simulink model "Channelizer_demo_panel"  (R2023b)
settings: Solver=VariableStepAuto  StartTime=0.0  StopTime=inf  RelTol=1e-3
PostLoadFcn:
  | TT = numerictype(1,16,15);
  | FF = fimath('RoundingMethod','Nearest','OverflowAction','Saturate');
  | mdl = channelizer_init(TT, FF);
  | channelizer = channelizer_model(mdl, TT, FF );
  | Ts = 16*(7/4)/8.75e9;
  | ch_filt_coef = rcosdesign(0.22,4,28,'normal');
  | ch_filt_coef = 28 * ch_filt_coef / sum(ch_filt_coef(:));
  | channelizer_demo_init;
values from neighbouring files (symbols this model uses):
  ch0_en = 0    [channelizer_demo_init.m]    (also in init.m)
  ch0_qam = 0    [channelizer_demo_init.m]    (also in init.m)
  ch0_swp = 0    [channelizer_demo_init.m]    (also in init.m)
  ch10_en = 0    [channelizer_demo_init.m]    (also in init.m)
  ch10_qam = 0    [channelizer_demo_init.m]    (also in init.m)
  ch10_swp = 0    [channelizer_demo_init.m]    (also in init.m)
  ch11_en = 0    [channelizer_demo_init.m]    (also in init.m)
  ch11_qam = 0    [channelizer_demo_init.m]    (also in init.m)
  ch11_swp = 0    [channelizer_demo_init.m]    (also in init.m)
  ch12_en = 0    [channelizer_demo_init.m]    (also in init.m)
  ch12_qam = 0    [channelizer_demo_init.m]    (also in init.m)
  ch12_swp = 0    [channelizer_demo_init.m]    (also in init.m)
  ch13_en = 0    [channelizer_demo_init.m]    (also in init.m)
  ch13_qam = 0    [channelizer_demo_init.m]    (also in init.m)
  ch13_swp = 0    [channelizer_demo_init.m]    (also in init.m)
  ch14_en = 0    [channelizer_demo_init.m]    (also in init.m)
  ch14_qam = 0    [channelizer_demo_init.m]    (also in init.m)
  ch14_swp = 0    [channelizer_demo_init.m]    (also in init.m)
  ch15_en = 0    [channelizer_demo_init.m]    (also in init.m)
  ch15_qam = 0    [channelizer_demo_init.m]    (also in init.m)
  ch15_swp = 0    [channelizer_demo_init.m]    (also in init.m)
  ch1_en = 1    [channelizer_demo_init.m]    (also in init.m)
  ch1_qam = 0    [channelizer_demo_init.m]    (also in init.m)
  ch1_swp = 0    [channelizer_demo_init.m]    (also in init.m)
  ch2_en = 1    [channelizer_demo_init.m]    (also in init.m)
  ch2_qam = 0    [channelizer_demo_init.m]    (also in init.m)
  ch2_swp = 0    [channelizer_demo_init.m]    (also in init.m)
  ch3_en = 0    [channelizer_demo_init.m]    (also in init.m)
  ch3_qam = 0    [channelizer_demo_init.m]    (also in init.m)
  ch3_swp = 0    [channelizer_demo_init.m]    (also in init.m)
  ch4_en = 0    [channelizer_demo_init.m]    (also in init.m)
  ch4_qam = 0    [channelizer_demo_init.m]    (also in init.m)
  ch4_swp = 0    [channelizer_demo_init.m]    (also in init.m)
  ch5_en = 1    [channelizer_demo_init.m]    (also in init.m)
  ch5_qam = 1    [channelizer_demo_init.m]    (also in init.m)
  ch5_swp = 0    [channelizer_demo_init.m]    (also in init.m)
  ch6_en = 1    [channelizer_demo_init.m]    (also in init.m)
  ch6_qam = 1    [channelizer_demo_init.m]    (also in init.m)
  ch6_swp = 0    [channelizer_demo_init.m]    (also in init.m)
  ch7_en = 0    [channelizer_demo_init.m]    (also in init.m)
  ch7_qam = 0    [channelizer_demo_init.m]    (also in init.m)
  ch7_swp = 0    [channelizer_demo_init.m]    (also in init.m)
  ch8_en = 0    [channelizer_demo_init.m]    (also in init.m)
  ch8_qam = 0    [channelizer_demo_init.m]    (also in init.m)
  ch8_swp = 0    [channelizer_demo_init.m]    (also in init.m)
  ch9_en = 0    [channelizer_demo_init.m]    (also in init.m)
  ch9_qam = 0    [channelizer_demo_init.m]    (also in init.m)
  ch9_swp = 0    [channelizer_demo_init.m]    (also in init.m)
  spec1_ch = 1    [channelizer_demo_init.m]    (also in init.m)
  spec2_ch = 2    [channelizer_demo_init.m]    (also in init.m)
  spec3_ch = 5    [channelizer_demo_init.m]    (also in init.m)
  spec4_ch = 6    [channelizer_demo_init.m]    (also in init.m)
  swp_rate0 = 0    [channelizer_demo_init.m]    (also in init.m)
  swp_rate1 = 0    [channelizer_demo_init.m]    (also in init.m)
  swp_rate10 = 0    [channelizer_demo_init.m]    (also in init.m)
  swp_rate11 = 0    [channelizer_demo_init.m]    (also in init.m)
  swp_rate12 = 0    [channelizer_demo_init.m]    (also in init.m)
  swp_rate13 = 0    [channelizer_demo_init.m]    (also in init.m)
  swp_rate14 = 0    [channelizer_demo_init.m]    (also in init.m)
  swp_rate15 = 0    [channelizer_demo_init.m]    (also in init.m)
  swp_rate2 = 0    [channelizer_demo_init.m]    (also in init.m)
  swp_rate3 = 0    [channelizer_demo_init.m]    (also in init.m)
  swp_rate4 = 0    [channelizer_demo_init.m]    (also in init.m)
  swp_rate5 = 0    [channelizer_demo_init.m]    (also in init.m)
  swp_rate6 = 0    [channelizer_demo_init.m]    (also in init.m)
  swp_rate7 = 0    [channelizer_demo_init.m]    (also in init.m)
  swp_rate8 = 0    [channelizer_demo_init.m]    (also in init.m)
  swp_rate9 = 0    [channelizer_demo_init.m]    (also in init.m)
undefined symbols (not defined in the file or in its folder): S, vsva2197, xcvc1902
libraries: aieUtilities x39, aieBasic x34, dspswit3 x16, dspsigops x16, hlsBasic x3, vmcUtilities x1, commchan3 x1
(part 3 of 5)

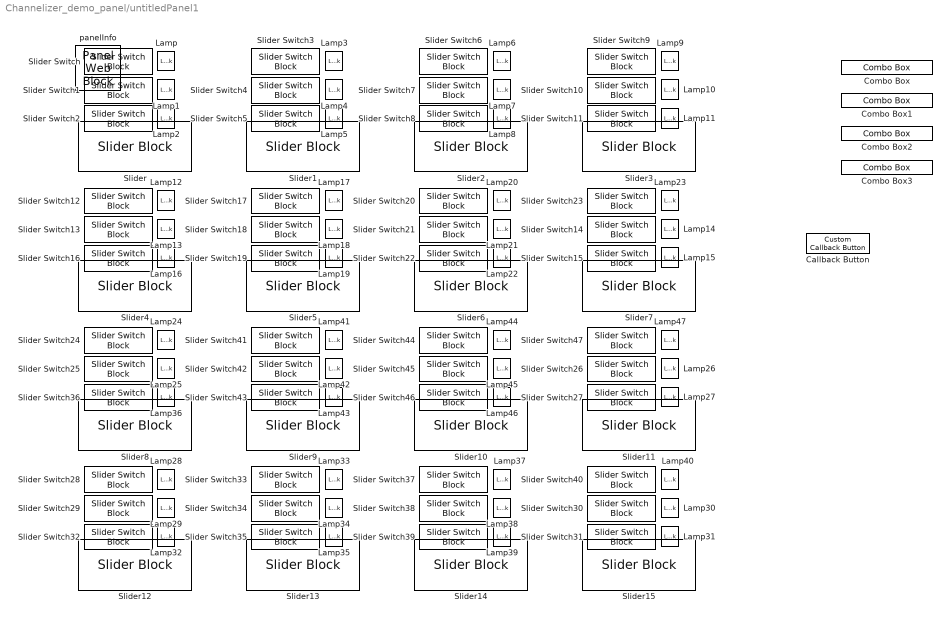
== system Channelizer_demo_panel/untitledPanel1 ==
  Callback Button : CustomCallbackButton  Tag=HiddenForWebPanel  PanelInfo="{\"addnFilesFolder\":\"\",\"height\":22,\"includeDebugPackages\":false,\"left\":833,\"outputFolder\":\"\",\"panelId\":\"panelId-6526f2f6-f2b9-454a-b79d-ddfd0d3181f7\",\"popoutMode\":\"\",\"standaloneTitle\":\"\",\"top\":225,\"type\":\"panelChild\",\"version\":\"2019b\",\"width\":70,\"zIndex\":1500128}"  Configuration="{\"components\":[{\"name\":\"BackgroundImageComponent\",\"settings\":{\"image\":{\"size\":[0,0],\"src\":\"default\",\"srcOrientation\":\"Right\"},\"position\":[0,0,1,1]}},{\"name\":\"ButtonStateComponent\",\"settings\":{\"buttonType\":\"momentary\",\"clickFcn\":\"channelizer_demo_init;\",\"onValue\":1,\"position\":[0,0,1,1],\"pressDelay\":\"500\",\"pressFcn\":\"\",\"repeatInterval\":\"0\",\"states\":[{\"horizontalAlignment\":\"center\",\"image\":{\"position\":[0,0,1,1],\"size\":[1,1],\"src\":\"default\",\"srcOrientation\":\"Right\"},\"label\":{\"color\":[1,1,1],\"icon\":{\"size\":[0,0],\"src\":\"default\",\"srcOrientation\":\"Right\"},\"iconPlacement\":\"left\",\"opacity\":1,\"show\":true,\"text\":{\"content\":\"RESET\",\"font\":\"Helvetica\",\"fontSize\":12}},\"labelOffset\":[0,0],\"verticalAlignment\":\"middle\"},{\"horizontalAlignment\":\"center\",\"image\":{\"position\":[0,0,1,1],\"size\":[1,1],\"src\":\"default\",\"srcOrientation\":\"Right\"},\"label\":{\"color\":[1,1,1],\"icon\":{\"size\":[0,0],\"src\":\"default\",\"srcOrientation\":\"Right\"},\"iconPlacement\":\"left\",\"opacity\":1,\"show\":true,\"text\":{\"content\":\"RESET\",\"font\":\"Helvetica\",\"fontSize\":12}},\"labelOffset\":[0,0],\"verticalAlignment\":\"middle\"},{\"horizontalAlignment\":\"center\",\"image\":{\"position\":[0,0,1,1],\"size\":[1,1],\"src\":\"default\",\"srcOrientation\":\"Right\"},\"label\":{\"color\":[1,1,1],\"icon\":{\"size\":[0,0],\"src\":\"default\",\"srcOrientation\":\"Right\"},\"iconPlacement\":\"left\",\"opacity\":1,\"show\":true,\"text\":{\"content\":\"RESET\",\"font\":\"Helvetica\",\"fontSize\":12}},\"labelOffset\":[0,0],\"verticalAlignment\":\"middle\"},{\"horizontalAlignment\":\"center\",\"image\":{\"position\":[0,0,1,1],\"size\":[1,1],\"src\":\"default\",\"srcOrientation\":\"Right\"},\"label\":{\"color\":[1,1,1],\"icon\":{\"size\":[0,0],\"src\":\"default\",\"srcOrientation\":\"Right\"},\"iconPlacement\":\"left\",\"opacity\":1,\"show\":true,\"text\":{\"content\":\"RESET\",\"font\":\"Helvetica\",\"fontSize\":12}},\"labelOffset\":[0,0],\"verticalAlignment\":\"middle\"}]}},{\"name\":\"ForegroundImageComponent\",\"settings\":{\"image\":{\"size\":[0,0],\"src\":\"default\",\"srcOrientation\":\"Right\"},\"isForeground\":1,\"position\":[0,0,1,1]}}],\"settings\":{\"BindingType\":\"standalone\",\"backgroundColor\":[244,244,244,1],\"backgroundOffset\":0.2,\"backgroundOpacity\":1,\"fixedAspectRatio\":\"on\",\"foregroundColor\":[0.01176470588,0.01176470588,0.01176470588,1],\"migratedFromLegacy\":true,\"useBackgroundColor\":true,\"variant\":\"callback\",\"version\":\"R2023a\"},\"type\":\"Button\"}"  CustomBackgroundColor="{\"color\":[0,0.447059,0.741176],\"show\":true}"
  Combo Box : ComboBox  Tag=HiddenForWebPanel  PanelInfo="{\"addnFilesFolder\":\"\",\"height\":16,\"includeDebugPackages\":false,\"left\":872,\"outputFolder\":\"\",\"panelId\":\"panelId-6526f2f6-f2b9-454a-b79d-ddfd0d3181f7\",\"popoutMode\":\"\",\"standaloneTitle\":\"\",\"top\":31,\"type\":\"panelChild\",\"version\":\"2019b\",\"width\":102,\"zIndex\":1500228}"  LabelPosition=Hide  SelectedLabel=Channel 1
      settings: Values={{'Channel 0', 'Channel 1', 'Channel 2', 'Channel 3', 'Channel 4', 'Channel 5', 'Channel 6', 'Channel 7', 'Channel 8', 'Channel 9', 'Channel 10', 'Channel 11', 'Channel 12', 'Channel 13', 'Channel 14', 'Channel 15'}, [0 1 2 3 4 5 6 7 8 9 10 11 12 13 14 15]}
  Combo Box1 : ComboBox  Tag=HiddenForWebPanel  PanelInfo="{\"addnFilesFolder\":\"\",\"height\":16,\"includeDebugPackages\":false,\"left\":872,\"outputFolder\":\"\",\"panelId\":\"panelId-6526f2f6-f2b9-454a-b79d-ddfd0d3181f7\",\"popoutMode\":\"\",\"standaloneTitle\":\"\",\"top\":68,\"type\":\"panelChild\",\"version\":\"2019b\",\"width\":102,\"zIndex\":1500208}"  LabelPosition=Hide  SelectedLabel=Channel 2
      settings: Values={{'Channel 0', 'Channel 1', 'Channel 2', 'Channel 3', 'Channel 4', 'Channel 5', 'Channel 6', 'Channel 7', 'Channel 8', 'Channel 9', 'Channel 10', 'Channel 11', 'Channel 12', 'Channel 13', 'Channel 14', 'Channel 15'}, [0 1 2 3 4 5 6 7 8 9 10 11 12 13 14 15]}
  Combo Box2 : ComboBox  Tag=HiddenForWebPanel  PanelInfo="{\"addnFilesFolder\":\"\",\"height\":16,\"includeDebugPackages\":false,\"left\":872,\"outputFolder\":\"\",\"panelId\":\"panelId-6526f2f6-f2b9-454a-b79d-ddfd0d3181f7\",\"popoutMode\":\"\",\"standaloneTitle\":\"\",\"top\":105,\"type\":\"panelChild\",\"version\":\"2019b\",\"width\":102,\"zIndex\":1500198}"  LabelPosition=Hide  SelectedLabel=Channel 5
      settings: Values={{'Channel 0', 'Channel 1', 'Channel 2', 'Channel 3', 'Channel 4', 'Channel 5', 'Channel 6', 'Channel 7', 'Channel 8', 'Channel 9', 'Channel 10', 'Channel 11', 'Channel 12', 'Channel 13', 'Channel 14', 'Channel 15'}, [0 1 2 3 4 5 6 7 8 9 10 11 12 13 14 15]}
  Combo Box3 : ComboBox  Tag=HiddenForWebPanel  PanelInfo="{\"addnFilesFolder\":\"\",\"height\":16,\"includeDebugPackages\":false,\"left\":872,\"outputFolder\":\"\",\"panelId\":\"panelId-6526f2f6-f2b9-454a-b79d-ddfd0d3181f7\",\"popoutMode\":\"\",\"standaloneTitle\":\"\",\"top\":143,\"type\":\"panelChild\",\"version\":\"2019b\",\"width\":102,\"zIndex\":1500096}"  LabelPosition=Hide  SelectedLabel=Channel 6
      settings: Values={{'Channel 0', 'Channel 1', 'Channel 2', 'Channel 3', 'Channel 4', 'Channel 5', 'Channel 6', 'Channel 7', 'Channel 8', 'Channel 9', 'Channel 10', 'Channel 11', 'Channel 12', 'Channel 13', 'Channel 14', 'Channel 15'}, [0 1 2 3 4 5 6 7 8 9 10 11 12 13 14 15]}
  Lamp : LampBlock  Tag=HiddenForWebPanel  PanelInfo="{\"addnFilesFolder\":\"\",\"height\":22,\"includeDebugPackages\":false,\"left\":107,\"outputFolder\":\"\",\"panelId\":\"panelId-6526f2f6-f2b9-454a-b79d-ddfd0d3181f7\",\"popoutMode\":\"\",\"standaloneTitle\":\"\",\"top\":21,\"type\":\"panelChild\",\"version\":\"2019b\",\"width\":19,\"zIndex\":1500094}"  LabelPosition=Hide
  Lamp1 : LampBlock  Tag=HiddenForWebPanel  PanelInfo="{\"addnFilesFolder\":\"\",\"height\":22,\"includeDebugPackages\":false,\"left\":107,\"outputFolder\":\"\",\"panelId\":\"panelId-6526f2f6-f2b9-454a-b79d-ddfd0d3181f7\",\"popoutMode\":\"\",\"standaloneTitle\":\"\",\"top\":53,\"type\":\"panelChild\",\"version\":\"2019b\",\"width\":19,\"zIndex\":1500030}"  LabelPosition=Hide
  Lamp10 : LampBlock  Tag=HiddenForWebPanel  PanelInfo="{\"addnFilesFolder\":\"\",\"height\":22,\"includeDebugPackages\":false,\"left\":671,\"outputFolder\":\"\",\"panelId\":\"panelId-6526f2f6-f2b9-454a-b79d-ddfd0d3181f7\",\"popoutMode\":\"\",\"standaloneTitle\":\"\",\"top\":53,\"type\":\"panelChild\",\"version\":\"2019b\",\"width\":19,\"zIndex\":1500212}"  LabelPosition=Hide
  Lamp11 : LampBlock  Tag=HiddenForWebPanel  PanelInfo="{\"addnFilesFolder\":\"\",\"height\":22,\"includeDebugPackages\":false,\"left\":671,\"outputFolder\":\"\",\"panelId\":\"panelId-6526f2f6-f2b9-454a-b79d-ddfd0d3181f7\",\"popoutMode\":\"\",\"standaloneTitle\":\"\",\"top\":85,\"type\":\"panelChild\",\"version\":\"2019b\",\"width\":19,\"zIndex\":1500102}"  LabelPosition=Hide
  Lamp12 : LampBlock  Tag=HiddenForWebPanel  PanelInfo="{\"addnFilesFolder\":\"\",\"height\":22,\"includeDebugPackages\":false,\"left\":107,\"outputFolder\":\"\",\"panelId\":\"panelId-6526f2f6-f2b9-454a-b79d-ddfd0d3181f7\",\"popoutMode\":\"\",\"standaloneTitle\":\"\",\"top\":177,\"type\":\"panelChild\",\"version\":\"2019b\",\"width\":19,\"zIndex\":1500110}"  LabelPosition=Hide
  Lamp13 : LampBlock  Tag=HiddenForWebPanel  PanelInfo="{\"addnFilesFolder\":\"\",\"height\":22,\"includeDebugPackages\":false,\"left\":107,\"outputFolder\":\"\",\"panelId\":\"panelId-6526f2f6-f2b9-454a-b79d-ddfd0d3181f7\",\"popoutMode\":\"\",\"standaloneTitle\":\"\",\"top\":209,\"type\":\"panelChild\",\"version\":\"2019b\",\"width\":19,\"zIndex\":1500034}"  LabelPosition=Hide
  Lamp14 : LampBlock  Tag=HiddenForWebPanel  PanelInfo="{\"addnFilesFolder\":\"\",\"height\":22,\"includeDebugPackages\":false,\"left\":671,\"outputFolder\":\"\",\"panelId\":\"panelId-6526f2f6-f2b9-454a-b79d-ddfd0d3181f7\",\"popoutMode\":\"\",\"standaloneTitle\":\"\",\"top\":209,\"type\":\"panelChild\",\"version\":\"2019b\",\"width\":19,\"zIndex\":1500166}"  LabelPosition=Hide
  Lamp15 : LampBlock  Tag=HiddenForWebPanel  PanelInfo="{\"addnFilesFolder\":\"\",\"height\":22,\"includeDebugPackages\":false,\"left\":671,\"outputFolder\":\"\",\"panelId\":\"panelId-6526f2f6-f2b9-454a-b79d-ddfd0d3181f7\",\"popoutMode\":\"\",\"standaloneTitle\":\"\",\"top\":241,\"type\":\"panelChild\",\"version\":\"2019b\",\"width\":19,\"zIndex\":1500042}"  LabelPosition=Hide
  Lamp16 : LampBlock  Tag=HiddenForWebPanel  PanelInfo="{\"addnFilesFolder\":\"\",\"height\":22,\"includeDebugPackages\":false,\"left\":107,\"outputFolder\":\"\",\"panelId\":\"panelId-6526f2f6-f2b9-454a-b79d-ddfd0d3181f7\",\"popoutMode\":\"\",\"standaloneTitle\":\"\",\"top\":241,\"type\":\"panelChild\",\"version\":\"2019b\",\"width\":19,\"zIndex\":1500210}"  LabelPosition=Hide
  Lamp17 : LampBlock  Tag=HiddenForWebPanel  PanelInfo="{\"addnFilesFolder\":\"\",\"height\":22,\"includeDebugPackages\":false,\"left\":295,\"outputFolder\":\"\",\"panelId\":\"panelId-6526f2f6-f2b9-454a-b79d-ddfd0d3181f7\",\"popoutMode\":\"\",\"standaloneTitle\":\"\",\"top\":177,\"type\":\"panelChild\",\"version\":\"2019b\",\"width\":19,\"zIndex\":1500108}"  LabelPosition=Hide
  Lamp18 : LampBlock  Tag=HiddenForWebPanel  PanelInfo="{\"addnFilesFolder\":\"\",\"height\":22,\"includeDebugPackages\":false,\"left\":295,\"outputFolder\":\"\",\"panelId\":\"panelId-6526f2f6-f2b9-454a-b79d-ddfd0d3181f7\",\"popoutMode\":\"\",\"standaloneTitle\":\"\",\"top\":209,\"type\":\"panelChild\",\"version\":\"2019b\",\"width\":19,\"zIndex\":1500200}"  LabelPosition=Hide
  Lamp19 : LampBlock  Tag=HiddenForWebPanel  PanelInfo="{\"addnFilesFolder\":\"\",\"height\":22,\"includeDebugPackages\":false,\"left\":295,\"outputFolder\":\"\",\"panelId\":\"panelId-6526f2f6-f2b9-454a-b79d-ddfd0d3181f7\",\"popoutMode\":\"\",\"standaloneTitle\":\"\",\"top\":241,\"type\":\"panelChild\",\"version\":\"2019b\",\"width\":19,\"zIndex\":1500188}"  LabelPosition=Hide
  Lamp2 : LampBlock  Tag=HiddenForWebPanel  PanelInfo="{\"addnFilesFolder\":\"\",\"height\":22,\"includeDebugPackages\":false,\"left\":107,\"outputFolder\":\"\",\"panelId\":\"panelId-6526f2f6-f2b9-454a-b79d-ddfd0d3181f7\",\"popoutMode\":\"\",\"standaloneTitle\":\"\",\"top\":85,\"type\":\"panelChild\",\"version\":\"2019b\",\"width\":19,\"zIndex\":1500028}"  LabelPosition=Hide
  Lamp20 : LampBlock  Tag=HiddenForWebPanel  PanelInfo="{\"addnFilesFolder\":\"\",\"height\":22,\"includeDebugPackages\":false,\"left\":483,\"outputFolder\":\"\",\"panelId\":\"panelId-6526f2f6-f2b9-454a-b79d-ddfd0d3181f7\",\"popoutMode\":\"\",\"standaloneTitle\":\"\",\"top\":177,\"type\":\"panelChild\",\"version\":\"2019b\",\"width\":19,\"zIndex\":1500116}"  LabelPosition=Hide
  Lamp21 : LampBlock  Tag=HiddenForWebPanel  PanelInfo="{\"addnFilesFolder\":\"\",\"height\":22,\"includeDebugPackages\":false,\"left\":483,\"outputFolder\":\"\",\"panelId\":\"panelId-6526f2f6-f2b9-454a-b79d-ddfd0d3181f7\",\"popoutMode\":\"\",\"standaloneTitle\":\"\",\"top\":209,\"type\":\"panelChild\",\"version\":\"2019b\",\"width\":19,\"zIndex\":1500072}"  LabelPosition=Hide
  Lamp22 : LampBlock  Tag=HiddenForWebPanel  PanelInfo="{\"addnFilesFolder\":\"\",\"height\":22,\"includeDebugPackages\":false,\"left\":483,\"outputFolder\":\"\",\"panelId\":\"panelId-6526f2f6-f2b9-454a-b79d-ddfd0d3181f7\",\"popoutMode\":\"\",\"standaloneTitle\":\"\",\"top\":241,\"type\":\"panelChild\",\"version\":\"2019b\",\"width\":19,\"zIndex\":1500046}"  LabelPosition=Hide
  Lamp23 : LampBlock  Tag=HiddenForWebPanel  PanelInfo="{\"addnFilesFolder\":\"\",\"height\":22,\"includeDebugPackages\":false,\"left\":671,\"outputFolder\":\"\",\"panelId\":\"panelId-6526f2f6-f2b9-454a-b79d-ddfd0d3181f7\",\"popoutMode\":\"\",\"standaloneTitle\":\"\",\"top\":177,\"type\":\"panelChild\",\"version\":\"2019b\",\"width\":19,\"zIndex\":1500004}"  LabelPosition=Hide
  Lamp24 : LampBlock  Tag=HiddenForWebPanel  PanelInfo="{\"addnFilesFolder\":\"\",\"height\":22,\"includeDebugPackages\":false,\"left\":107,\"outputFolder\":\"\",\"panelId\":\"panelId-6526f2f6-f2b9-454a-b79d-ddfd0d3181f7\",\"popoutMode\":\"\",\"standaloneTitle\":\"\",\"top\":333,\"type\":\"panelChild\",\"version\":\"2019b\",\"width\":19,\"zIndex\":1500078}"  LabelPosition=Hide
  Lamp25 : LampBlock  Tag=HiddenForWebPanel  PanelInfo="{\"addnFilesFolder\":\"\",\"height\":22,\"includeDebugPackages\":false,\"left\":107,\"outputFolder\":\"\",\"panelId\":\"panelId-6526f2f6-f2b9-454a-b79d-ddfd0d3181f7\",\"popoutMode\":\"\",\"standaloneTitle\":\"\",\"top\":365,\"type\":\"panelChild\",\"version\":\"2019b\",\"width\":19,\"zIndex\":1500038}"  LabelPosition=Hide
  Lamp26 : LampBlock  Tag=HiddenForWebPanel  PanelInfo="{\"addnFilesFolder\":\"\",\"height\":22,\"includeDebugPackages\":false,\"left\":671,\"outputFolder\":\"\",\"panelId\":\"panelId-6526f2f6-f2b9-454a-b79d-ddfd0d3181f7\",\"popoutMode\":\"\",\"standaloneTitle\":\"\",\"top\":365,\"type\":\"panelChild\",\"version\":\"2019b\",\"width\":19,\"zIndex\":1500158}"  LabelPosition=Hide
  Lamp27 : LampBlock  Tag=HiddenForWebPanel  PanelInfo="{\"addnFilesFolder\":\"\",\"height\":22,\"includeDebugPackages\":false,\"left\":671,\"outputFolder\":\"\",\"panelId\":\"panelId-6526f2f6-f2b9-454a-b79d-ddfd0d3181f7\",\"popoutMode\":\"\",\"standaloneTitle\":\"\",\"top\":397,\"type\":\"panelChild\",\"version\":\"2019b\",\"width\":19,\"zIndex\":1500024}"  LabelPosition=Hide
  Lamp28 : LampBlock  Tag=HiddenForWebPanel  PanelInfo="{\"addnFilesFolder\":\"\",\"height\":22,\"includeDebugPackages\":false,\"left\":107,\"outputFolder\":\"\",\"panelId\":\"panelId-6526f2f6-f2b9-454a-b79d-ddfd0d3181f7\",\"popoutMode\":\"\",\"standaloneTitle\":\"\",\"top\":489,\"type\":\"panelChild\",\"version\":\"2019b\",\"width\":19,\"zIndex\":1500134}"  LabelPosition=Hide
  Lamp29 : LampBlock  Tag=HiddenForWebPanel  PanelInfo="{\"addnFilesFolder\":\"\",\"height\":22,\"includeDebugPackages\":false,\"left\":107,\"outputFolder\":\"\",\"panelId\":\"panelId-6526f2f6-f2b9-454a-b79d-ddfd0d3181f7\",\"popoutMode\":\"\",\"standaloneTitle\":\"\",\"top\":521,\"type\":\"panelChild\",\"version\":\"2019b\",\"width\":19,\"zIndex\":1500080}"  LabelPosition=Hide
  Lamp3 : LampBlock  Tag=HiddenForWebPanel  PanelInfo="{\"addnFilesFolder\":\"\",\"height\":22,\"includeDebugPackages\":false,\"left\":295,\"outputFolder\":\"\",\"panelId\":\"panelId-6526f2f6-f2b9-454a-b79d-ddfd0d3181f7\",\"popoutMode\":\"\",\"standaloneTitle\":\"\",\"top\":21,\"type\":\"panelChild\",\"version\":\"2019b\",\"width\":19,\"zIndex\":1500056}"  LabelPosition=Hide
  Lamp30 : LampBlock  Tag=HiddenForWebPanel  PanelInfo="{\"addnFilesFolder\":\"\",\"height\":22,\"includeDebugPackages\":false,\"left\":671,\"outputFolder\":\"\",\"panelId\":\"panelId-6526f2f6-f2b9-454a-b79d-ddfd0d3181f7\",\"popoutMode\":\"\",\"standaloneTitle\":\"\",\"top\":521,\"type\":\"panelChild\",\"version\":\"2019b\",\"width\":19,\"zIndex\":1500186}"  LabelPosition=Hide
  Lamp31 : LampBlock  Tag=HiddenForWebPanel  PanelInfo="{\"addnFilesFolder\":\"\",\"height\":22,\"includeDebugPackages\":false,\"left\":671,\"outputFolder\":\"\",\"panelId\":\"panelId-6526f2f6-f2b9-454a-b79d-ddfd0d3181f7\",\"popoutMode\":\"\",\"standaloneTitle\":\"\",\"top\":553,\"type\":\"panelChild\",\"version\":\"2019b\",\"width\":19,\"zIndex\":1500050}"  LabelPosition=Hide
  Lamp32 : LampBlock  Tag=HiddenForWebPanel  PanelInfo="{\"addnFilesFolder\":\"\",\"height\":22,\"includeDebugPackages\":false,\"left\":107,\"outputFolder\":\"\",\"panelId\":\"panelId-6526f2f6-f2b9-454a-b79d-ddfd0d3181f7\",\"popoutMode\":\"\",\"standaloneTitle\":\"\",\"top\":553,\"type\":\"panelChild\",\"version\":\"2019b\",\"width\":19,\"zIndex\":1500088}"  LabelPosition=Hide
  Lamp33 : LampBlock  Tag=HiddenForWebPanel  PanelInfo="{\"addnFilesFolder\":\"\",\"height\":22,\"includeDebugPackages\":false,\"left\":295,\"outputFolder\":\"\",\"panelId\":\"panelId-6526f2f6-f2b9-454a-b79d-ddfd0d3181f7\",\"popoutMode\":\"\",\"standaloneTitle\":\"\",\"top\":489,\"type\":\"panelChild\",\"version\":\"2019b\",\"width\":19,\"zIndex\":1500086}"  LabelPosition=Hide
  Lamp34 : LampBlock  Tag=HiddenForWebPanel  PanelInfo="{\"addnFilesFolder\":\"\",\"height\":22,\"includeDebugPackages\":false,\"left\":295,\"outputFolder\":\"\",\"panelId\":\"panelId-6526f2f6-f2b9-454a-b79d-ddfd0d3181f7\",\"popoutMode\":\"\",\"standaloneTitle\":\"\",\"top\":521,\"type\":\"panelChild\",\"version\":\"2019b\",\"width\":19,\"zIndex\":1500098}"  LabelPosition=Hide
  Lamp35 : LampBlock  Tag=HiddenForWebPanel  PanelInfo="{\"addnFilesFolder\":\"\",\"height\":22,\"includeDebugPackages\":false,\"left\":295,\"outputFolder\":\"\",\"panelId\":\"panelId-6526f2f6-f2b9-454a-b79d-ddfd0d3181f7\",\"popoutMode\":\"\",\"standaloneTitle\":\"\",\"top\":553,\"type\":\"panelChild\",\"version\":\"2019b\",\"width\":19,\"zIndex\":1500100}"  LabelPosition=Hide
  Lamp36 : LampBlock  Tag=HiddenForWebPanel  PanelInfo="{\"addnFilesFolder\":\"\",\"height\":22,\"includeDebugPackages\":false,\"left\":107,\"outputFolder\":\"\",\"panelId\":\"panelId-6526f2f6-f2b9-454a-b79d-ddfd0d3181f7\",\"popoutMode\":\"\",\"standaloneTitle\":\"\",\"top\":397,\"type\":\"panelChild\",\"version\":\"2019b\",\"width\":19,\"zIndex\":1500140}"  LabelPosition=Hide
  Lamp37 : LampBlock  Tag=HiddenForWebPanel  PanelInfo="{\"addnFilesFolder\":\"\",\"height\":22,\"includeDebugPackages\":false,\"left\":483,\"outputFolder\":\"\",\"panelId\":\"panelId-6526f2f6-f2b9-454a-b79d-ddfd0d3181f7\",\"popoutMode\":\"\",\"standaloneTitle\":\"\",\"top\":489,\"type\":\"panelChild\",\"version\":\"2019b\",\"width\":19,\"zIndex\":1500138}"  LabelPosition=Hide
  Lamp38 : LampBlock  Tag=HiddenForWebPanel  PanelInfo="{\"addnFilesFolder\":\"\",\"height\":22,\"includeDebugPackages\":false,\"left\":483,\"outputFolder\":\"\",\"panelId\":\"panelId-6526f2f6-f2b9-454a-b79d-ddfd0d3181f7\",\"popoutMode\":\"\",\"standaloneTitle\":\"\",\"top\":521,\"type\":\"panelChild\",\"version\":\"2019b\",\"width\":19,\"zIndex\":1500206}"  LabelPosition=Hide
  Lamp39 : LampBlock  Tag=HiddenForWebPanel  PanelInfo="{\"addnFilesFolder\":\"\",\"height\":22,\"includeDebugPackages\":false,\"left\":483,\"outputFolder\":\"\",\"panelId\":\"panelId-6526f2f6-f2b9-454a-b79d-ddfd0d3181f7\",\"popoutMode\":\"\",\"standaloneTitle\":\"\",\"top\":553,\"type\":\"panelChild\",\"version\":\"2019b\",\"width\":19,\"zIndex\":1500130}"  LabelPosition=Hide
  Lamp4 : LampBlock  Tag=HiddenForWebPanel  PanelInfo="{\"addnFilesFolder\":\"\",\"height\":22,\"includeDebugPackages\":false,\"left\":295,\"outputFolder\":\"\",\"panelId\":\"panelId-6526f2f6-f2b9-454a-b79d-ddfd0d3181f7\",\"popoutMode\":\"\",\"standaloneTitle\":\"\",\"top\":53,\"type\":\"panelChild\",\"version\":\"2019b\",\"width\":19,\"zIndex\":1500054}"  LabelPosition=Hide
  Lamp40 : LampBlock  Tag=HiddenForWebPanel  PanelInfo="{\"addnFilesFolder\":\"\",\"height\":22,\"includeDebugPackages\":false,\"left\":671,\"outputFolder\":\"\",\"panelId\":\"panelId-6526f2f6-f2b9-454a-b79d-ddfd0d3181f7\",\"popoutMode\":\"\",\"standaloneTitle\":\"\",\"top\":489,\"type\":\"panelChild\",\"version\":\"2019b\",\"width\":19,\"zIndex\":1500016}"  LabelPosition=Hide
  Lamp41 : LampBlock  Tag=HiddenForWebPanel  PanelInfo="{\"addnFilesFolder\":\"\",\"height\":22,\"includeDebugPackages\":false,\"left\":295,\"outputFolder\":\"\",\"panelId\":\"panelId-6526f2f6-f2b9-454a-b79d-ddfd0d3181f7\",\"popoutMode\":\"\",\"standaloneTitle\":\"\",\"top\":333,\"type\":\"panelChild\",\"version\":\"2019b\",\"width\":19,\"zIndex\":1500068}"  LabelPosition=Hide
  Lamp42 : LampBlock  Tag=HiddenForWebPanel  PanelInfo="{\"addnFilesFolder\":\"\",\"height\":22,\"includeDebugPackages\":false,\"left\":295,\"outputFolder\":\"\",\"panelId\":\"panelId-6526f2f6-f2b9-454a-b79d-ddfd0d3181f7\",\"popoutMode\":\"\",\"standaloneTitle\":\"\",\"top\":365,\"type\":\"panelChild\",\"version\":\"2019b\",\"width\":19,\"zIndex\":1500076}"  LabelPosition=Hide
  Lamp43 : LampBlock  Tag=HiddenForWebPanel  PanelInfo="{\"addnFilesFolder\":\"\",\"height\":22,\"includeDebugPackages\":false,\"left\":295,\"outputFolder\":\"\",\"panelId\":\"panelId-6526f2f6-f2b9-454a-b79d-ddfd0d3181f7\",\"popoutMode\":\"\",\"standaloneTitle\":\"\",\"top\":397,\"type\":\"panelChild\",\"version\":\"2019b\",\"width\":19,\"zIndex\":1500084}"  LabelPosition=Hide
  Lamp44 : LampBlock  Tag=HiddenForWebPanel  PanelInfo="{\"addnFilesFolder\":\"\",\"height\":22,\"includeDebugPackages\":false,\"left\":483,\"outputFolder\":\"\",\"panelId\":\"panelId-6526f2f6-f2b9-454a-b79d-ddfd0d3181f7\",\"popoutMode\":\"\",\"standaloneTitle\":\"\",\"top\":333,\"type\":\"panelChild\",\"version\":\"2019b\",\"width\":19,\"zIndex\":1500124}"  LabelPosition=Hide
  Lamp45 : LampBlock  Tag=HiddenForWebPanel  PanelInfo="{\"addnFilesFolder\":\"\",\"height\":22,\"includeDebugPackages\":false,\"left\":483,\"outputFolder\":\"\",\"panelId\":\"panelId-6526f2f6-f2b9-454a-b79d-ddfd0d3181f7\",\"popoutMode\":\"\",\"standaloneTitle\":\"\",\"top\":365,\"type\":\"panelChild\",\"version\":\"2019b\",\"width\":19,\"zIndex\":1500164}"  LabelPosition=Hide
  Lamp46 : LampBlock  Tag=HiddenForWebPanel  PanelInfo="{\"addnFilesFolder\":\"\",\"height\":22,\"includeDebugPackages\":false,\"left\":483,\"outputFolder\":\"\",\"panelId\":\"panelId-6526f2f6-f2b9-454a-b79d-ddfd0d3181f7\",\"popoutMode\":\"\",\"standaloneTitle\":\"\",\"top\":397,\"type\":\"panelChild\",\"version\":\"2019b\",\"width\":19,\"zIndex\":1500132}"  LabelPosition=Hide
  Lamp47 : LampBlock  Tag=HiddenForWebPanel  PanelInfo="{\"addnFilesFolder\":\"\",\"height\":22,\"includeDebugPackages\":false,\"left\":671,\"outputFolder\":\"\",\"panelId\":\"panelId-6526f2f6-f2b9-454a-b79d-ddfd0d3181f7\",\"popoutMode\":\"\",\"standaloneTitle\":\"\",\"top\":333,\"type\":\"panelChild\",\"version\":\"2019b\",\"width\":19,\"zIndex\":1500126}"  LabelPosition=Hide
  Lamp5 : LampBlock  Tag=HiddenForWebPanel  PanelInfo="{\"addnFilesFolder\":\"\",\"height\":22,\"includeDebugPackages\":false,\"left\":295,\"outputFolder\":\"\",\"panelId\":\"panelId-6526f2f6-f2b9-454a-b79d-ddfd0d3181f7\",\"popoutMode\":\"\",\"standaloneTitle\":\"\",\"top\":85,\"type\":\"panelChild\",\"version\":\"2019b\",\"width\":19,\"zIndex\":1500022}"  LabelPosition=Hide
  Lamp6 : LampBlock  Tag=HiddenForWebPanel  PanelInfo="{\"addnFilesFolder\":\"\",\"height\":22,\"includeDebugPackages\":false,\"left\":483,\"outputFolder\":\"\",\"panelId\":\"panelId-6526f2f6-f2b9-454a-b79d-ddfd0d3181f7\",\"popoutMode\":\"\",\"standaloneTitle\":\"\",\"top\":21,\"type\":\"panelChild\",\"version\":\"2019b\",\"width\":19,\"zIndex\":1500044}"  LabelPosition=Hide
  Lamp7 : LampBlock  Tag=HiddenForWebPanel  PanelInfo="{\"addnFilesFolder\":\"\",\"height\":22,\"includeDebugPackages\":false,\"left\":483,\"outputFolder\":\"\",\"panelId\":\"panelId-6526f2f6-f2b9-454a-b79d-ddfd0d3181f7\",\"popoutMode\":\"\",\"standaloneTitle\":\"\",\"top\":53,\"type\":\"panelChild\",\"version\":\"2019b\",\"width\":19,\"zIndex\":1500018}"  LabelPosition=Hide
  Lamp8 : LampBlock  Tag=HiddenForWebPanel  PanelInfo="{\"addnFilesFolder\":\"\",\"height\":22,\"includeDebugPackages\":false,\"left\":483,\"outputFolder\":\"\",\"panelId\":\"panelId-6526f2f6-f2b9-454a-b79d-ddfd0d3181f7\",\"popoutMode\":\"\",\"standaloneTitle\":\"\",\"top\":85,\"type\":\"panelChild\",\"version\":\"2019b\",\"width\":19,\"zIndex\":1500092}"  LabelPosition=Hide
  Lamp9 : LampBlock  Tag=HiddenForWebPanel  PanelInfo="{\"addnFilesFolder\":\"\",\"height\":22,\"includeDebugPackages\":false,\"left\":671,\"outputFolder\":\"\",\"panelId\":\"panelId-6526f2f6-f2b9-454a-b79d-ddfd0d3181f7\",\"popoutMode\":\"\",\"standaloneTitle\":\"\",\"top\":21,\"type\":\"panelChild\",\"version\":\"2019b\",\"width\":19,\"zIndex\":1500032}"  LabelPosition=Hide
  Slider : SliderBlock  Tag=HiddenForWebPanel  PanelInfo="{\"addnFilesFolder\":\"\",\"height\":57,\"includeDebugPackages\":false,\"left\":18,\"outputFolder\":\"\",\"panelId\":\"panelId-6526f2f6-f2b9-454a-b79d-ddfd0d3181f7\",\"popoutMode\":\"\",\"standaloneTitle\":\"\",\"top\":99,\"type\":\"panelChild\",\"version\":\"2019b\",\"width\":127,\"zIndex\":1500222}"  LabelPosition=Hide  ScaleMin=-0.1  ScaleMax=0.1
  Slider Switch : SliderSwitchBlock  Tag=HiddenForWebPanel  PanelInfo="{\"addnFilesFolder\":\"\",\"height\":29,\"includeDebugPackages\":false,\"left\":25,\"outputFolder\":\"\",\"panelId\":\"panelId-6526f2f6-f2b9-454a-b79d-ddfd0d3181f7\",\"popoutMode\":\"\",\"standaloneTitle\":\"\",\"top\":18,\"type\":\"panelChild\",\"version\":\"2019b\",\"width\":76,\"zIndex\":1500074}"  LabelPosition=Hide
      settings: Values={{'Off', 'On'}, [0 1]}
  Slider Switch1 : SliderSwitchBlock  Tag=HiddenForWebPanel  PanelInfo="{\"addnFilesFolder\":\"\",\"height\":29,\"includeDebugPackages\":false,\"left\":25,\"outputFolder\":\"\",\"panelId\":\"panelId-6526f2f6-f2b9-454a-b79d-ddfd0d3181f7\",\"popoutMode\":\"\",\"standaloneTitle\":\"\",\"top\":50,\"type\":\"panelChild\",\"version\":\"2019b\",\"width\":76,\"zIndex\":1500150}"  LabelPosition=Hide
      settings: Values={{'Off', 'On'}, [0 1]}
  Slider Switch10 : SliderSwitchBlock  Tag=HiddenForWebPanel  PanelInfo="{\"addnFilesFolder\":\"\",\"height\":29,\"includeDebugPackages\":false,\"left\":588,\"outputFolder\":\"\",\"panelId\":\"panelId-6526f2f6-f2b9-454a-b79d-ddfd0d3181f7\",\"popoutMode\":\"\",\"standaloneTitle\":\"\",\"top\":50,\"type\":\"panelChild\",\"version\":\"2019b\",\"width\":76,\"zIndex\":1500180}"  LabelPosition=Hide
      settings: Values={{'Off', 'On'}, [0 1]}
  Slider Switch11 : SliderSwitchBlock  Tag=HiddenForWebPanel  PanelInfo="{\"addnFilesFolder\":\"\",\"height\":29,\"includeDebugPackages\":false,\"left\":588,\"outputFolder\":\"\",\"panelId\":\"panelId-6526f2f6-f2b9-454a-b79d-ddfd0d3181f7\",\"popoutMode\":\"\",\"standaloneTitle\":\"\",\"top\":82,\"type\":\"panelChild\",\"version\":\"2019b\",\"width\":76,\"zIndex\":1500082}"  LabelPosition=Hide
      settings: Values={{'Off', 'On'}, [0 1]}
  Slider Switch12 : SliderSwitchBlock  Tag=HiddenForWebPanel  PanelInfo="{\"addnFilesFolder\":\"\",\"height\":29,\"includeDebugPackages\":false,\"left\":25,\"outputFolder\":\"\",\"panelId\":\"panelId-6526f2f6-f2b9-454a-b79d-ddfd0d3181f7\",\"popoutMode\":\"\",\"standaloneTitle\":\"\",\"top\":174,\"type\":\"panelChild\",\"version\":\"2019b\",\"width\":76,\"zIndex\":1500152}"  LabelPosition=Hide
      settings: Values={{'Off', 'On'}, [0 1]}
  Slider Switch13 : SliderSwitchBlock  Tag=HiddenForWebPanel  PanelInfo="{\"addnFilesFolder\":\"\",\"height\":29,\"includeDebugPackages\":false,\"left\":25,\"outputFolder\":\"\",\"panelId\":\"panelId-6526f2f6-f2b9-454a-b79d-ddfd0d3181f7\",\"popoutMode\":\"\",\"standaloneTitle\":\"\",\"top\":206,\"type\":\"panelChild\",\"version\":\"2019b\",\"width\":76,\"zIndex\":1500120}"  LabelPosition=Hide
      settings: Values={{'Off', 'On'}, [0 1]}
  Slider Switch14 : SliderSwitchBlock  Tag=HiddenForWebPanel  PanelInfo="{\"addnFilesFolder\":\"\",\"height\":29,\"includeDebugPackages\":false,\"left\":588,\"outputFolder\":\"\",\"panelId\":\"panelId-6526f2f6-f2b9-454a-b79d-ddfd0d3181f7\",\"popoutMode\":\"\",\"standaloneTitle\":\"\",\"top\":206,\"type\":\"panelChild\",\"version\":\"2019b\",\"width\":76,\"zIndex\":1500008}"  LabelPosition=Hide
      settings: Values={{'Off', 'On'}, [0 1]}
  Slider Switch15 : SliderSwitchBlock  Tag=HiddenForWebPanel  PanelInfo="{\"addnFilesFolder\":\"\",\"height\":29,\"includeDebugPackages\":false,\"left\":588,\"outputFolder\":\"\",\"panelId\":\"panelId-6526f2f6-f2b9-454a-b79d-ddfd0d3181f7\",\"popoutMode\":\"\",\"standaloneTitle\":\"\",\"top\":238,\"type\":\"panelChild\",\"version\":\"2019b\",\"width\":76,\"zIndex\":1500226}"  LabelPosition=Hide
      settings: Values={{'Off', 'On'}, [0 1]}
  Slider Switch16 : SliderSwitchBlock  Tag=HiddenForWebPanel  PanelInfo="{\"addnFilesFolder\":\"\",\"height\":29,\"includeDebugPackages\":false,\"left\":25,\"outputFolder\":\"\",\"panelId\":\"panelId-6526f2f6-f2b9-454a-b79d-ddfd0d3181f7\",\"popoutMode\":\"\",\"standaloneTitle\":\"\",\"top\":238,\"type\":\"panelChild\",\"version\":\"2019b\",\"width\":76,\"zIndex\":1500176}"  LabelPosition=Hide
      settings: Values={{'Off', 'On'}, [0 1]}
  Slider Switch17 : SliderSwitchBlock  Tag=HiddenForWebPanel  PanelInfo="{\"addnFilesFolder\":\"\",\"height\":29,\"includeDebugPackages\":false,\"left\":212,\"outputFolder\":\"\",\"panelId\":\"panelId-6526f2f6-f2b9-454a-b79d-ddfd0d3181f7\",\"popoutMode\":\"\",\"standaloneTitle\":\"\",\"top\":174,\"type\":\"panelChild\",\"version\":\"2019b\",\"width\":76,\"zIndex\":1500020}"  LabelPosition=Hide
      settings: Values={{'Off', 'On'}, [0 1]}
  Slider Switch18 : SliderSwitchBlock  Tag=HiddenForWebPanel  PanelInfo="{\"addnFilesFolder\":\"\",\"height\":29,\"includeDebugPackages\":false,\"left\":212,\"outputFolder\":\"\",\"panelId\":\"panelId-6526f2f6-f2b9-454a-b79d-ddfd0d3181f7\",\"popoutMode\":\"\",\"standaloneTitle\":\"\",\"top\":206,\"type\":\"panelChild\",\"version\":\"2019b\",\"width\":76,\"zIndex\":1500192}"  LabelPosition=Hide
      settings: Values={{'Off', 'On'}, [0 1]}
  Slider Switch19 : SliderSwitchBlock  Tag=HiddenForWebPanel  PanelInfo="{\"addnFilesFolder\":\"\",\"height\":29,\"includeDebugPackages\":false,\"left\":212,\"outputFolder\":\"\",\"panelId\":\"panelId-6526f2f6-f2b9-454a-b79d-ddfd0d3181f7\",\"popoutMode\":\"\",\"standaloneTitle\":\"\",\"top\":238,\"type\":\"panelChild\",\"version\":\"2019b\",\"width\":76,\"zIndex\":1500052}"  LabelPosition=Hide
      settings: Values={{'Off', 'On'}, [0 1]}
  Slider Switch2 : SliderSwitchBlock  Tag=HiddenForWebPanel  PanelInfo="{\"addnFilesFolder\":\"\",\"height\":29,\"includeDebugPackages\":false,\"left\":25,\"outputFolder\":\"\",\"panelId\":\"panelId-6526f2f6-f2b9-454a-b79d-ddfd0d3181f7\",\"popoutMode\":\"\",\"standaloneTitle\":\"\",\"top\":82,\"type\":\"panelChild\",\"version\":\"2019b\",\"width\":76,\"zIndex\":1500066}"  LabelPosition=Hide
      settings: Values={{'Off', 'On'}, [0 1]}
  Slider Switch20 : SliderSwitchBlock  Tag=HiddenForWebPanel  PanelInfo="{\"addnFilesFolder\":\"\",\"height\":29,\"includeDebugPackages\":false,\"left\":400,\"outputFolder\":\"\",\"panelId\":\"panelId-6526f2f6-f2b9-454a-b79d-ddfd0d3181f7\",\"popoutMode\":\"\",\"standaloneTitle\":\"\",\"top\":174,\"type\":\"panelChild\",\"version\":\"2019b\",\"width\":76,\"zIndex\":1500058}"  LabelPosition=Hide
      settings: Values={{'Off', 'On'}, [0 1]}
  Slider Switch21 : SliderSwitchBlock  Tag=HiddenForWebPanel  PanelInfo="{\"addnFilesFolder\":\"\",\"height\":29,\"includeDebugPackages\":false,\"left\":400,\"outputFolder\":\"\",\"panelId\":\"panelId-6526f2f6-f2b9-454a-b79d-ddfd0d3181f7\",\"popoutMode\":\"\",\"standaloneTitle\":\"\",\"top\":206,\"type\":\"panelChild\",\"version\":\"2019b\",\"width\":76,\"zIndex\":1500012}"  LabelPosition=Hide
      settings: Values={{'Off', 'On'}, [0 1]}
  Slider Switch22 : SliderSwitchBlock  Tag=HiddenForWebPanel  PanelInfo="{\"addnFilesFolder\":\"\",\"height\":29,\"includeDebugPackages\":false,\"left\":400,\"outputFolder\":\"\",\"panelId\":\"panelId-6526f2f6-f2b9-454a-b79d-ddfd0d3181f7\",\"popoutMode\":\"\",\"standaloneTitle\":\"\",\"top\":238,\"type\":\"panelChild\",\"version\":\"2019b\",\"width\":76,\"zIndex\":1500112}"  LabelPosition=Hide
      settings: Values={{'Off', 'On'}, [0 1]}
  Slider Switch23 : SliderSwitchBlock  Tag=HiddenForWebPanel  PanelInfo="{\"addnFilesFolder\":\"\",\"height\":29,\"includeDebugPackages\":false,\"left\":588,\"outputFolder\":\"\",\"panelId\":\"panelId-6526f2f6-f2b9-454a-b79d-ddfd0d3181f7\",\"popoutMode\":\"\",\"standaloneTitle\":\"\",\"top\":174,\"type\":\"panelChild\",\"version\":\"2019b\",\"width\":76,\"zIndex\":1500014}"  LabelPosition=Hide
      settings: Values={{'Off', 'On'}, [0 1]}
  Slider Switch24 : SliderSwitchBlock  Tag=HiddenForWebPanel  PanelInfo="{\"addnFilesFolder\":\"\",\"height\":29,\"includeDebugPackages\":false,\"left\":25,\"outputFolder\":\"\",\"panelId\":\"panelId-6526f2f6-f2b9-454a-b79d-ddfd0d3181f7\",\"popoutMode\":\"\",\"standaloneTitle\":\"\",\"top\":330,\"type\":\"panelChild\",\"version\":\"2019b\",\"width\":76,\"zIndex\":1500122}"  LabelPosition=Hide
      settings: Values={{'Off', 'On'}, [0 1]}
  Slider Switch25 : SliderSwitchBlock  Tag=HiddenForWebPanel  PanelInfo="{\"addnFilesFolder\":\"\",\"height\":29,\"includeDebugPackages\":false,\"left\":25,\"outputFolder\":\"\",\"panelId\":\"panelId-6526f2f6-f2b9-454a-b79d-ddfd0d3181f7\",\"popoutMode\":\"\",\"standaloneTitle\":\"\",\"top\":362,\"type\":\"panelChild\",\"version\":\"2019b\",\"width\":76,\"zIndex\":1500118}"  LabelPosition=Hide
      settings: Values={{'Off', 'On'}, [0 1]}
  Slider Switch26 : SliderSwitchBlock  Tag=HiddenForWebPanel  PanelInfo="{\"addnFilesFolder\":\"\",\"height\":29,\"includeDebugPackages\":false,\"left\":588,\"outputFolder\":\"\",\"panelId\":\"panelId-6526f2f6-f2b9-454a-b79d-ddfd0d3181f7\",\"popoutMode\":\"\",\"standaloneTitle\":\"\",\"top\":362,\"type\":\"panelChild\",\"version\":\"2019b\",\"width\":76,\"zIndex\":1500154}"  LabelPosition=Hide
      settings: Values={{'Off', 'On'}, [0 1]}
  Slider Switch27 : SliderSwitchBlock  Tag=HiddenForWebPanel  PanelInfo="{\"addnFilesFolder\":\"\",\"height\":29,\"includeDebugPackages\":false,\"left\":588,\"outputFolder\":\"\",\"panelId\":\"panelId-6526f2f6-f2b9-454a-b79d-ddfd0d3181f7\",\"popoutMode\":\"\",\"standaloneTitle\":\"\",\"top\":394,\"type\":\"panelChild\",\"version\":\"2019b\",\"width\":76,\"zIndex\":1500148}"  LabelPosition=Hide
      settings: Values={{'Off', 'On'}, [0 1]}
  Slider Switch28 : SliderSwitchBlock  Tag=HiddenForWebPanel  PanelInfo="{\"addnFilesFolder\":\"\",\"height\":29,\"includeDebugPackages\":false,\"left\":25,\"outputFolder\":\"\",\"panelId\":\"panelId-6526f2f6-f2b9-454a-b79d-ddfd0d3181f7\",\"popoutMode\":\"\",\"standaloneTitle\":\"\",\"top\":486,\"type\":\"panelChild\",\"version\":\"2019b\",\"width\":76,\"zIndex\":1500178}"  LabelPosition=Hide
      settings: Values={{'Off', 'On'}, [0 1]}
  Slider Switch29 : SliderSwitchBlock  Tag=HiddenForWebPanel  PanelInfo="{\"addnFilesFolder\":\"\",\"height\":29,\"includeDebugPackages\":false,\"left\":25,\"outputFolder\":\"\",\"panelId\":\"panelId-6526f2f6-f2b9-454a-b79d-ddfd0d3181f7\",\"popoutMode\":\"\",\"standaloneTitle\":\"\",\"top\":518,\"type\":\"panelChild\",\"version\":\"2019b\",\"width\":76,\"zIndex\":1500232}"  LabelPosition=Hide
      settings: Values={{'Off', 'On'}, [0 1]}
  Slider Switch3 : SliderSwitchBlock  Tag=HiddenForWebPanel  PanelInfo="{\"addnFilesFolder\":\"\",\"height\":29,\"includeDebugPackages\":false,\"left\":212,\"outputFolder\":\"\",\"panelId\":\"panelId-6526f2f6-f2b9-454a-b79d-ddfd0d3181f7\",\"popoutMode\":\"\",\"standaloneTitle\":\"\",\"top\":18,\"type\":\"panelChild\",\"version\":\"2019b\",\"width\":76,\"zIndex\":1500006}"  LabelPosition=Hide
      settings: Values={{'Off', 'On'}, [0 1]}
  Slider Switch30 : SliderSwitchBlock  Tag=HiddenForWebPanel  PanelInfo="{\"addnFilesFolder\":\"\",\"height\":29,\"includeDebugPackages\":false,\"left\":588,\"outputFolder\":\"\",\"panelId\":\"panelId-6526f2f6-f2b9-454a-b79d-ddfd0d3181f7\",\"popoutMode\":\"\",\"standaloneTitle\":\"\",\"top\":518,\"type\":\"panelChild\",\"version\":\"2019b\",\"width\":76,\"zIndex\":1500190}"  LabelPosition=Hide
      settings: Values={{'Off', 'On'}, [0 1]}
  Slider Switch31 : SliderSwitchBlock  Tag=HiddenForWebPanel  PanelInfo="{\"addnFilesFolder\":\"\",\"height\":29,\"includeDebugPackages\":false,\"left\":588,\"outputFolder\":\"\",\"panelId\":\"panelId-6526f2f6-f2b9-454a-b79d-ddfd0d3181f7\",\"popoutMode\":\"\",\"standaloneTitle\":\"\",\"top\":550,\"type\":\"panelChild\",\"version\":\"2019b\",\"width\":76,\"zIndex\":1500114}"  LabelPosition=Hide
      settings: Values={{'Off', 'On'}, [0 1]}
  Slider Switch32 : SliderSwitchBlock  Tag=HiddenForWebPanel  PanelInfo="{\"addnFilesFolder\":\"\",\"height\":29,\"includeDebugPackages\":false,\"left\":25,\"outputFolder\":\"\",\"panelId\":\"panelId-6526f2f6-f2b9-454a-b79d-ddfd0d3181f7\",\"popoutMode\":\"\",\"standaloneTitle\":\"\",\"top\":550,\"type\":\"panelChild\",\"version\":\"2019b\",\"width\":76,\"zIndex\":1500204}"  LabelPosition=Hide
      settings: Values={{'Off', 'On'}, [0 1]}
  Slider Switch33 : SliderSwitchBlock  Tag=HiddenForWebPanel  PanelInfo="{\"addnFilesFolder\":\"\",\"height\":29,\"includeDebugPackages\":false,\"left\":212,\"outputFolder\":\"\",\"panelId\":\"panelId-6526f2f6-f2b9-454a-b79d-ddfd0d3181f7\",\"popoutMode\":\"\",\"standaloneTitle\":\"\",\"top\":486,\"type\":\"panelChild\",\"version\":\"2019b\",\"width\":76,\"zIndex\":1500062}"  LabelPosition=Hide
      settings: Values={{'Off', 'On'}, [0 1]}
  Slider Switch34 : SliderSwitchBlock  Tag=HiddenForWebPanel  PanelInfo="{\"addnFilesFolder\":\"\",\"height\":29,\"includeDebugPackages\":false,\"left\":212,\"outputFolder\":\"\",\"panelId\":\"panelId-6526f2f6-f2b9-454a-b79d-ddfd0d3181f7\",\"popoutMode\":\"\",\"standaloneTitle\":\"\",\"top\":518,\"type\":\"panelChild\",\"version\":\"2019b\",\"width\":76,\"zIndex\":1500026}"  LabelPosition=Hide
      settings: Values={{'Off', 'On'}, [0 1]}
  Slider Switch35 : SliderSwitchBlock  Tag=HiddenForWebPanel  PanelInfo="{\"addnFilesFolder\":\"\",\"height\":29,\"includeDebugPackages\":false,\"left\":212,\"outputFolder\":\"\",\"panelId\":\"panelId-6526f2f6-f2b9-454a-b79d-ddfd0d3181f7\",\"popoutMode\":\"\",\"standaloneTitle\":\"\",\"top\":550,\"type\":\"panelChild\",\"version\":\"2019b\",\"width\":76,\"zIndex\":1500196}"  LabelPosition=Hide
      settings: Values={{'Off', 'On'}, [0 1]}
  Slider Switch36 : SliderSwitchBlock  Tag=HiddenForWebPanel  PanelInfo="{\"addnFilesFolder\":\"\",\"height\":29,\"includeDebugPackages\":false,\"left\":25,\"outputFolder\":\"\",\"panelId\":\"panelId-6526f2f6-f2b9-454a-b79d-ddfd0d3181f7\",\"popoutMode\":\"\",\"standaloneTitle\":\"\",\"top\":394,\"type\":\"panelChild\",\"version\":\"2019b\",\"width\":76,\"zIndex\":1500162}"  LabelPosition=Hide
      settings: Values={{'Off', 'On'}, [0 1]}
  Slider Switch37 : SliderSwitchBlock  Tag=HiddenForWebPanel  PanelInfo="{\"addnFilesFolder\":\"\",\"height\":29,\"includeDebugPackages\":false,\"left\":400,\"outputFolder\":\"\",\"panelId\":\"panelId-6526f2f6-f2b9-454a-b79d-ddfd0d3181f7\",\"popoutMode\":\"\",\"standaloneTitle\":\"\",\"top\":486,\"type\":\"panelChild\",\"version\":\"2019b\",\"width\":76,\"zIndex\":1500168}"  LabelPosition=Hide
      settings: Values={{'Off', 'On'}, [0 1]}
  Slider Switch38 : SliderSwitchBlock  Tag=HiddenForWebPanel  PanelInfo="{\"addnFilesFolder\":\"\",\"height\":29,\"includeDebugPackages\":false,\"left\":400,\"outputFolder\":\"\",\"panelId\":\"panelId-6526f2f6-f2b9-454a-b79d-ddfd0d3181f7\",\"popoutMode\":\"\",\"standaloneTitle\":\"\",\"top\":518,\"type\":\"panelChild\",\"version\":\"2019b\",\"width\":76,\"zIndex\":1500202}"  LabelPosition=Hide
      settings: Values={{'Off', 'On'}, [0 1]}
  Slider Switch39 : SliderSwitchBlock  Tag=HiddenForWebPanel  PanelInfo="{\"addnFilesFolder\":\"\",\"height\":29,\"includeDebugPackages\":false,\"left\":400,\"outputFolder\":\"\",\"panelId\":\"panelId-6526f2f6-f2b9-454a-b79d-ddfd0d3181f7\",\"popoutMode\":\"\",\"standaloneTitle\":\"\",\"top\":550,\"type\":\"panelChild\",\"version\":\"2019b\",\"width\":76,\"zIndex\":1500064}"  LabelPosition=Hide
      settings: Values={{'Off', 'On'}, [0 1]}
  Slider Switch4 : SliderSwitchBlock  Tag=HiddenForWebPanel  PanelInfo="{\"addnFilesFolder\":\"\",\"height\":29,\"includeDebugPackages\":false,\"left\":212,\"outputFolder\":\"\",\"panelId\":\"panelId-6526f2f6-f2b9-454a-b79d-ddfd0d3181f7\",\"popoutMode\":\"\",\"standaloneTitle\":\"\",\"top\":50,\"type\":\"panelChild\",\"version\":\"2019b\",\"width\":76,\"zIndex\":1500136}"  LabelPosition=Hide
      settings: Values={{'Off', 'On'}, [0 1]}
  Slider Switch40 : SliderSwitchBlock  Tag=HiddenForWebPanel  PanelInfo="{\"addnFilesFolder\":\"\",\"height\":29,\"includeDebugPackages\":false,\"left\":588,\"outputFolder\":\"\",\"panelId\":\"panelId-6526f2f6-f2b9-454a-b79d-ddfd0d3181f7\",\"popoutMode\":\"\",\"standaloneTitle\":\"\",\"top\":486,\"type\":\"panelChild\",\"version\":\"2019b\",\"width\":76,\"zIndex\":1500220}"  LabelPosition=Hide
      settings: Values={{'Off', 'On'}, [0 1]}
  Slider Switch41 : SliderSwitchBlock  Tag=HiddenForWebPanel  PanelInfo="{\"addnFilesFolder\":\"\",\"height\":29,\"includeDebugPackages\":false,\"left\":212,\"outputFolder\":\"\",\"panelId\":\"panelId-6526f2f6-f2b9-454a-b79d-ddfd0d3181f7\",\"popoutMode\":\"\",\"standaloneTitle\":\"\",\"top\":330,\"type\":\"panelChild\",\"version\":\"2019b\",\"width\":76,\"zIndex\":1500214}"  LabelPosition=Hide
      settings: Values={{'Off', 'On'}, [0 1]}
  Slider Switch42 : SliderSwitchBlock  Tag=HiddenForWebPanel  PanelInfo="{\"addnFilesFolder\":\"\",\"height\":29,\"includeDebugPackages\":false,\"left\":212,\"outputFolder\":\"\",\"panelId\":\"panelId-6526f2f6-f2b9-454a-b79d-ddfd0d3181f7\",\"popoutMode\":\"\",\"standaloneTitle\":\"\",\"top\":362,\"type\":\"panelChild\",\"version\":\"2019b\",\"width\":76,\"zIndex\":1500172}"  LabelPosition=Hide
      settings: Values={{'Off', 'On'}, [0 1]}
  Slider Switch43 : SliderSwitchBlock  Tag=HiddenForWebPanel  PanelInfo="{\"addnFilesFolder\":\"\",\"height\":29,\"includeDebugPackages\":false,\"left\":212,\"outputFolder\":\"\",\"panelId\":\"panelId-6526f2f6-f2b9-454a-b79d-ddfd0d3181f7\",\"popoutMode\":\"\",\"standaloneTitle\":\"\",\"top\":394,\"type\":\"panelChild\",\"version\":\"2019b\",\"width\":76,\"zIndex\":1500156}"  LabelPosition=Hide
      settings: Values={{'Off', 'On'}, [0 1]}
  Slider Switch44 : SliderSwitchBlock  Tag=HiddenForWebPanel  PanelInfo="{\"addnFilesFolder\":\"\",\"height\":29,\"includeDebugPackages\":false,\"left\":400,\"outputFolder\":\"\",\"panelId\":\"panelId-6526f2f6-f2b9-454a-b79d-ddfd0d3181f7\",\"popoutMode\":\"\",\"standaloneTitle\":\"\",\"top\":330,\"type\":\"panelChild\",\"version\":\"2019b\",\"width\":76,\"zIndex\":1500060}"  LabelPosition=Hide
      settings: Values={{'Off', 'On'}, [0 1]}
  Slider Switch45 : SliderSwitchBlock  Tag=HiddenForWebPanel  PanelInfo="{\"addnFilesFolder\":\"\",\"height\":29,\"includeDebugPackages\":false,\"left\":400,\"outputFolder\":\"\",\"panelId\":\"panelId-6526f2f6-f2b9-454a-b79d-ddfd0d3181f7\",\"popoutMode\":\"\",\"standaloneTitle\":\"\",\"top\":362,\"type\":\"panelChild\",\"version\":\"2019b\",\"width\":76,\"zIndex\":1500146}"  LabelPosition=Hide
      settings: Values={{'Off', 'On'}, [0 1]}
  Slider Switch46 : SliderSwitchBlock  Tag=HiddenForWebPanel  PanelInfo="{\"addnFilesFolder\":\"\",\"height\":29,\"includeDebugPackages\":false,\"left\":400,\"outputFolder\":\"\",\"panelId\":\"panelId-6526f2f6-f2b9-454a-b79d-ddfd0d3181f7\",\"popoutMode\":\"\",\"standaloneTitle\":\"\",\"top\":394,\"type\":\"panelChild\",\"version\":\"2019b\",\"width\":76,\"zIndex\":1500218}"  LabelPosition=Hide
      settings: Values={{'Off', 'On'}, [0 1]}
  Slider Switch47 : SliderSwitchBlock  Tag=HiddenForWebPanel  PanelInfo="{\"addnFilesFolder\":\"\",\"height\":29,\"includeDebugPackages\":false,\"left\":588,\"outputFolder\":\"\",\"panelId\":\"panelId-6526f2f6-f2b9-454a-b79d-ddfd0d3181f7\",\"popoutMode\":\"\",\"standaloneTitle\":\"\",\"top\":330,\"type\":\"panelChild\",\"version\":\"2019b\",\"width\":76,\"zIndex\":1500104}"  LabelPosition=Hide
      settings: Values={{'Off', 'On'}, [0 1]}
  Slider Switch5 : SliderSwitchBlock  Tag=HiddenForWebPanel  PanelInfo="{\"addnFilesFolder\":\"\",\"height\":29,\"includeDebugPackages\":false,\"left\":212,\"outputFolder\":\"\",\"panelId\":\"panelId-6526f2f6-f2b9-454a-b79d-ddfd0d3181f7\",\"popoutMode\":\"\",\"standaloneTitle\":\"\",\"top\":82,\"type\":\"panelChild\",\"version\":\"2019b\",\"width\":76,\"zIndex\":1500174}"  LabelPosition=Hide
      settings: Values={{'Off', 'On'}, [0 1]}
  Slider Switch6 : SliderSwitchBlock  Tag=HiddenForWebPanel  PanelInfo="{\"addnFilesFolder\":\"\",\"height\":29,\"includeDebugPackages\":false,\"left\":400,\"outputFolder\":\"\",\"panelId\":\"panelId-6526f2f6-f2b9-454a-b79d-ddfd0d3181f7\",\"popoutMode\":\"\",\"standaloneTitle\":\"\",\"top\":18,\"type\":\"panelChild\",\"version\":\"2019b\",\"width\":76,\"zIndex\":1500230}"  LabelPosition=Hide
      settings: Values={{'Off', 'On'}, [0 1]}
  Slider Switch7 : SliderSwitchBlock  Tag=HiddenForWebPanel  PanelInfo="{\"addnFilesFolder\":\"\",\"height\":29,\"includeDebugPackages\":false,\"left\":400,\"outputFolder\":\"\",\"panelId\":\"panelId-6526f2f6-f2b9-454a-b79d-ddfd0d3181f7\",\"popoutMode\":\"\",\"standaloneTitle\":\"\",\"top\":50,\"type\":\"panelChild\",\"version\":\"2019b\",\"width\":76,\"zIndex\":1500170}"  LabelPosition=Hide
      settings: Values={{'Off', 'On'}, [0 1]}
  Slider Switch8 : SliderSwitchBlock  Tag=HiddenForWebPanel  PanelInfo="{\"addnFilesFolder\":\"\",\"height\":29,\"includeDebugPackages\":false,\"left\":400,\"outputFolder\":\"\",\"panelId\":\"panelId-6526f2f6-f2b9-454a-b79d-ddfd0d3181f7\",\"popoutMode\":\"\",\"standaloneTitle\":\"\",\"top\":82,\"type\":\"panelChild\",\"version\":\"2019b\",\"width\":76,\"zIndex\":1500216}"  LabelPosition=Hide
      settings: Values={{'Off', 'On'}, [0 1]}
  Slider Switch9 : SliderSwitchBlock  Tag=HiddenForWebPanel  PanelInfo="{\"addnFilesFolder\":\"\",\"height\":29,\"includeDebugPackages\":false,\"left\":588,\"outputFolder\":\"\",\"panelId\":\"panelId-6526f2f6-f2b9-454a-b79d-ddfd0d3181f7\",\"popoutMode\":\"\",\"standaloneTitle\":\"\",\"top\":18,\"type\":\"panelChild\",\"version\":\"2019b\",\"width\":76,\"zIndex\":1500142}"  LabelPosition=Hide
      settings: Values={{'Off', 'On'}, [0 1]}
  Slider1 : SliderBlock  Tag=HiddenForWebPanel  PanelInfo="{\"addnFilesFolder\":\"\",\"height\":57,\"includeDebugPackages\":false,\"left\":206,\"outputFolder\":\"\",\"panelId\":\"panelId-6526f2f6-f2b9-454a-b79d-ddfd0d3181f7\",\"popoutMode\":\"\",\"standaloneTitle\":\"\",\"top\":99,\"type\":\"panelChild\",\"version\":\"2019b\",\"width\":127,\"zIndex\":1500010}"  LabelPosition=Hide  ScaleMin=-0.1  ScaleMax=0.1
  Slider10 : SliderBlock  Tag=HiddenForWebPanel  PanelInfo="{\"addnFilesFolder\":\"\",\"height\":57,\"includeDebugPackages\":false,\"left\":394,\"outputFolder\":\"\",\"panelId\":\"panelId-6526f2f6-f2b9-454a-b79d-ddfd0d3181f7\",\"popoutMode\":\"\",\"standaloneTitle\":\"\",\"top\":411,\"type\":\"panelChild\",\"version\":\"2019b\",\"width\":127,\"zIndex\":1500182}"  LabelPosition=Hide  ScaleMin=-1  ScaleMax=1
  Slider11 : SliderBlock  Tag=HiddenForWebPanel  PanelInfo="{\"addnFilesFolder\":\"\",\"height\":57,\"includeDebugPackages\":false,\"left\":582,\"outputFolder\":\"\",\"panelId\":\"panelId-6526f2f6-f2b9-454a-b79d-ddfd0d3181f7\",\"popoutMode\":\"\",\"standaloneTitle\":\"\",\"top\":411,\"type\":\"panelChild\",\"version\":\"2019b\",\"width\":127,\"zIndex\":1500002}"  LabelPosition=Hide  ScaleMin=-1  ScaleMax=1
  Slider12 : SliderBlock  Tag=HiddenForWebPanel  PanelInfo="{\"addnFilesFolder\":\"\",\"height\":57,\"includeDebugPackages\":false,\"left\":18,\"outputFolder\":\"\",\"panelId\":\"panelId-6526f2f6-f2b9-454a-b79d-ddfd0d3181f7\",\"popoutMode\":\"\",\"standaloneTitle\":\"\",\"top\":567,\"type\":\"panelChild\",\"version\":\"2019b\",\"width\":127,\"zIndex\":1500090}"  LabelPosition=Hide  ScaleMin=-5  ScaleMax=5
  Slider13 : SliderBlock  Tag=HiddenForWebPanel  PanelInfo="{\"addnFilesFolder\":\"\",\"height\":57,\"includeDebugPackages\":false,\"left\":206,\"outputFolder\":\"\",\"panelId\":\"panelId-6526f2f6-f2b9-454a-b79d-ddfd0d3181f7\",\"popoutMode\":\"\",\"standaloneTitle\":\"\",\"top\":567,\"type\":\"panelChild\",\"version\":\"2019b\",\"width\":127,\"zIndex\":1500144}"  LabelPosition=Hide  ScaleMin=-5  ScaleMax=5
  Slider14 : SliderBlock  Tag=HiddenForWebPanel  PanelInfo="{\"addnFilesFolder\":\"\",\"height\":57,\"includeDebugPackages\":false,\"left\":394,\"outputFolder\":\"\",\"panelId\":\"panelId-6526f2f6-f2b9-454a-b79d-ddfd0d3181f7\",\"popoutMode\":\"\",\"standaloneTitle\":\"\",\"top\":567,\"type\":\"panelChild\",\"version\":\"2019b\",\"width\":127,\"zIndex\":1500184}"  LabelPosition=Hide  ScaleMin=-5  ScaleMax=5
  Slider15 : SliderBlock  Tag=HiddenForWebPanel  PanelInfo="{\"addnFilesFolder\":\"\",\"height\":57,\"includeDebugPackages\":false,\"left\":582,\"outputFolder\":\"\",\"panelId\":\"panelId-6526f2f6-f2b9-454a-b79d-ddfd0d3181f7\",\"popoutMode\":\"\",\"standaloneTitle\":\"\",\"top\":567,\"type\":\"panelChild\",\"version\":\"2019b\",\"width\":127,\"zIndex\":1500234}"  LabelPosition=Hide  ScaleMin=-5  ScaleMax=5
  Slider2 : SliderBlock  Tag=HiddenForWebPanel  PanelInfo="{\"addnFilesFolder\":\"\",\"height\":57,\"includeDebugPackages\":false,\"left\":394,\"outputFolder\":\"\",\"panelId\":\"panelId-6526f2f6-f2b9-454a-b79d-ddfd0d3181f7\",\"popoutMode\":\"\",\"standaloneTitle\":\"\",\"top\":99,\"type\":\"panelChild\",\"version\":\"2019b\",\"width\":127,\"zIndex\":1500040}"  LabelPosition=Hide  ScaleMin=-0.1  ScaleMax=0.1
  Slider3 : SliderBlock  Tag=HiddenForWebPanel  PanelInfo="{\"addnFilesFolder\":\"\",\"height\":57,\"includeDebugPackages\":false,\"left\":582,\"outputFolder\":\"\",\"panelId\":\"panelId-6526f2f6-f2b9-454a-b79d-ddfd0d3181f7\",\"popoutMode\":\"\",\"standaloneTitle\":\"\",\"top\":99,\"type\":\"panelChild\",\"version\":\"2019b\",\"width\":127,\"zIndex\":1500036}"  LabelPosition=Hide  ScaleMin=-0.1  ScaleMax=0.1
  Slider4 : SliderBlock  Tag=HiddenForWebPanel  PanelInfo="{\"addnFilesFolder\":\"\",\"height\":57,\"includeDebugPackages\":false,\"left\":18,\"outputFolder\":\"\",\"panelId\":\"panelId-6526f2f6-f2b9-454a-b79d-ddfd0d3181f7\",\"popoutMode\":\"\",\"standaloneTitle\":\"\",\"top\":255,\"type\":\"panelChild\",\"version\":\"2019b\",\"width\":127,\"zIndex\":1500194}"  LabelPosition=Hide  ScaleMin=-0.5  ScaleMax=0.5
  Slider5 : SliderBlock  Tag=HiddenForWebPanel  PanelInfo="{\"addnFilesFolder\":\"\",\"height\":57,\"includeDebugPackages\":false,\"left\":206,\"outputFolder\":\"\",\"panelId\":\"panelId-6526f2f6-f2b9-454a-b79d-ddfd0d3181f7\",\"popoutMode\":\"\",\"standaloneTitle\":\"\",\"top\":255,\"type\":\"panelChild\",\"version\":\"2019b\",\"width\":127,\"zIndex\":1500070}"  LabelPosition=Hide  ScaleMin=-0.5  ScaleMax=0.5
  Slider6 : SliderBlock  Tag=HiddenForWebPanel  PanelInfo="{\"addnFilesFolder\":\"\",\"height\":57,\"includeDebugPackages\":false,\"left\":394,\"outputFolder\":\"\",\"panelId\":\"panelId-6526f2f6-f2b9-454a-b79d-ddfd0d3181f7\",\"popoutMode\":\"\",\"standaloneTitle\":\"\",\"top\":255,\"type\":\"panelChild\",\"version\":\"2019b\",\"width\":127,\"zIndex\":1500160}"  LabelPosition=Hide  ScaleMin=-0.5  ScaleMax=0.5
  Slider7 : SliderBlock  Tag=HiddenForWebPanel  PanelInfo="{\"addnFilesFolder\":\"\",\"height\":57,\"includeDebugPackages\":false,\"left\":582,\"outputFolder\":\"\",\"panelId\":\"panelId-6526f2f6-f2b9-454a-b79d-ddfd0d3181f7\",\"popoutMode\":\"\",\"standaloneTitle\":\"\",\"top\":255,\"type\":\"panelChild\",\"version\":\"2019b\",\"width\":127,\"zIndex\":1500106}"  LabelPosition=Hide  ScaleMin=-0.5  ScaleMax=0.5
  Slider8 : SliderBlock  Tag=HiddenForWebPanel  PanelInfo="{\"addnFilesFolder\":\"\",\"height\":57,\"includeDebugPackages\":false,\"left\":18,\"outputFolder\":\"\",\"panelId\":\"panelId-6526f2f6-f2b9-454a-b79d-ddfd0d3181f7\",\"popoutMode\":\"\",\"standaloneTitle\":\"\",\"top\":411,\"type\":\"panelChild\",\"version\":\"2019b\",\"width\":127,\"zIndex\":1500224}"  LabelPosition=Hide  ScaleMin=-1  ScaleMax=1
  Slider9 : SliderBlock  Tag=HiddenForWebPanel  PanelInfo="{\"addnFilesFolder\":\"\",\"height\":57,\"includeDebugPackages\":false,\"left\":206,\"outputFolder\":\"\",\"panelId\":\"panelId-6526f2f6-f2b9-454a-b79d-ddfd0d3181f7\",\"popoutMode\":\"\",\"standaloneTitle\":\"\",\"top\":411,\"type\":\"panelChild\",\"version\":\"2019b\",\"width\":127,\"zIndex\":1500048}"  LabelPosition=Hide  ScaleMin=-1  ScaleMax=1
  panelInfo : PanelWebBlock  Tag=HiddenForWebPanel  PanelInfo="{\"addnFilesFolder\":\"\",\"compacted\":false,\"height\":646,\"includeDebugPackages\":false,\"isActiveTab\":true,\"left\":58,\"name\":\"Panel1\",\"outputFolder\":\"\",\"panelId\":\"panelId-6526f2f6-f2b9-454a-b79d-ddfd0d3181f7\",\"popoutMode\":\"\",\"standaloneTitle\":\"\",\"tabIndex\":0,\"tabbedSetId\":\"tabbedSet7455043051\",\"top\":28,\"type\":\"panel\",\"version\":\"2019b\",\"visible\":true,\"width\":996,\"zIndex\":1500004}"
